simulink model "control"  (R2020a)
settings: Solver=VariableStepAuto  StartTime=0.0  StopTime=10.0  RelTol=1e-3
values from neighbouring files (symbols this model uses):
  A_m = [ 0 1 0; M_alpha 0 M_alpha/V ... (first row only)    [State_space.m]
  B_m = [0; M_delta; Tc/m ]    [State_space.m]
  C_m = diag([1 1 1])    [State_space.m]
  D_m = [0;0;0]    [State_space.m]
  K_1 = K(1)    [Cost_function.m]
  K_2 = K(2)    [Cost_function.m]
  K_3 = K(3)    [Cost_function.m]
settings Model: Creator=Edd.ie  LastModifiedBy=Edd.ie

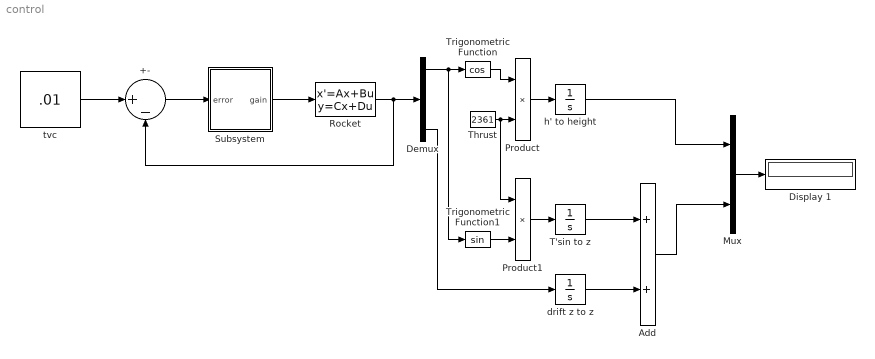
== system control ==
  +- : Sum  Inputs=|+-
  Add : Sum
  Demux : Demux  Outputs=3
  Display 1 : Display
  Mux : Mux  Inputs=2
  Product : Product
  Product1 : Product
  Rocket : StateSpace  A=A_m  B=B_m  C=C_m  D=D_m  InitialCondition=[0.2;0;0]
  Subsystem : Subsystem
  T'sin to z : Integrator
  Thrust : Constant  Value=2361
  Trigonometric Function : Trigonometry  Operator=cos
  Trigonometric Function1 : Trigonometry
  drift z to z : Integrator
  h' to height : Integrator
  tvc : Constant  Value=.01
  wires:
  tvc/1 -> +-/1
  +-/1 -> Subsystem/1(error)
  Subsystem/1(gain) -> Rocket/1
  Rocket/1 -> +-/2, Demux/1
  Demux/1 -> Trigonometric Function1/1, Trigonometric Function/1
  Trigonometric Function/1 -> Product/1
  Thrust/1 -> Product1/1, Product/2
  Trigonometric Function1/1 -> Product1/2
  Demux/3 -> drift z to z/1
  Product1/1 -> T'sin to z/1
  T'sin to z/1 -> Add/1
  drift z to z/1 -> Add/2
  Product/1 -> h' to height/1
  Mux/1 -> Display 1/1
  Add/1 -> Mux/2
  h' to height/1 -> Mux/1

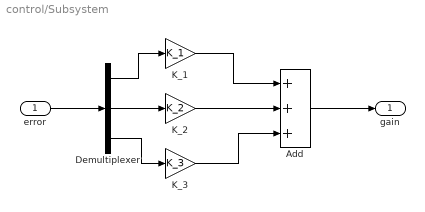
== system control/Subsystem ==
  error : Inport
  Add : Sum  Inputs=+++
  Demultiplexer : Demux  Outputs=3
  K_1 : Gain  Gain=K_1
  K_2 : Gain  Gain=K_2
  K_3 : Gain  Gain=K_3
  gain : Outport
  wires:
  K_1/1 -> Add/1
  Add/1 -> gain/1
  Demultiplexer/1 -> K_1/1
  K_2/1 -> Add/2
  Demultiplexer/3 -> K_3/1
  error/1 -> Demultiplexer/1
  Demultiplexer/2 -> K_2/1
  K_3/1 -> Add/3
